simulink model "exp1"  (R2021b)
settings: Solver=VariableStepAuto  StartTime=0.0  StopTime=10.0  RelTol=1e-3
settings Model: Creator=ashir  LastModifiedBy=ashir

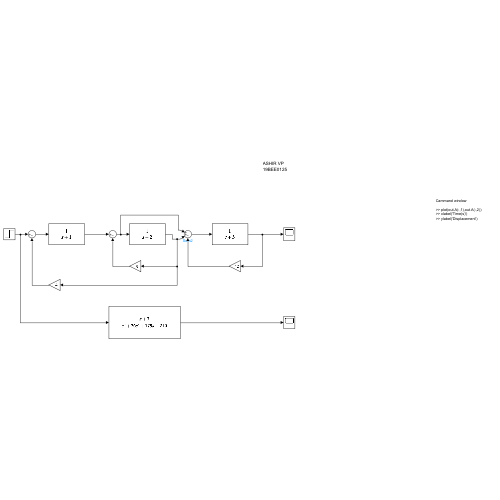
[thumbnail: Simulink's stored preview of the top-level diagram]
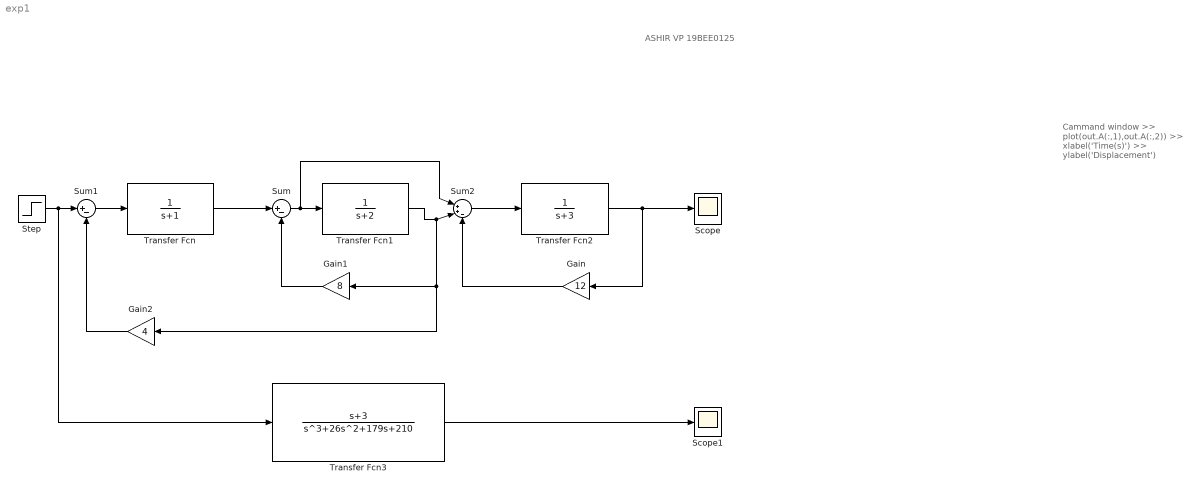
== system exp1 ==
  note: Cammand window
      |
      | >> plot(out.A(:,1),out.A(:,2))
      | >> xlabel('Time(s)')
      | >> ylabel('Displacement')
  note: ASHIR VP
      | 19BEE0125
  Gain : Gain  Gain=12
  Gain1 : Gain  Gain=8
  Gain2 : Gain  Gain=4
  Scope : Scope
  Scope1 : Scope
  Step : Step  Time=0  SampleTime=0
  Sum : Sum  Inputs=|+-
  Sum1 : Sum  Inputs=|+-
  Sum2 : Sum  Inputs=|++-
  Transfer Fcn : TransferFcn  Denominator=[1 1]
  Transfer Fcn1 : TransferFcn  Denominator=[1 2]
  Transfer Fcn2 : TransferFcn  Denominator=[1 3]
  Transfer Fcn3 : TransferFcn  Numerator=[1 3]  Denominator=[1 26 179 210]
  wires:
  Step/1 -> Transfer Fcn3/1, Sum1/1
  Sum1/1 -> Transfer Fcn/1
  Transfer Fcn/1 -> Sum/1
  Sum/1 -> Sum2/1, Transfer Fcn1/1
  Transfer Fcn1/1 -> Gain2/1, Gain1/1, Sum2/2
  Transfer Fcn2/1 -> Gain/1, Scope/1
  Sum2/1 -> Transfer Fcn2/1
  Gain/1 -> Sum2/3
  Gain1/1 -> Sum/2
  Gain2/1 -> Sum1/2
  Transfer Fcn3/1 -> Scope1/1
